simulink model "AMCLIB_CurrentLoop_BAM_FLT"  (Simulink 8.3)
settings: Solver=ode45  StartTime=0.0  StopTime=10.0  RelTol=1e-3
undefined symbols (not defined in the file): fltCC1scD, fltCC1scQ, fltCC2scD, fltCC2scQ
settings Model: Creator=B37097  LastModifiedBy=B37097
settings DataIOCC: SignalLoggingSaveFormat=Dataset
settings DebuggingCC: UnderspecifiedInitializationDetection=Simplified  StateNameClashWarn=none
settings GRTTargetCC: CombineOutputUpdateFcns=on  GRTInterface=off

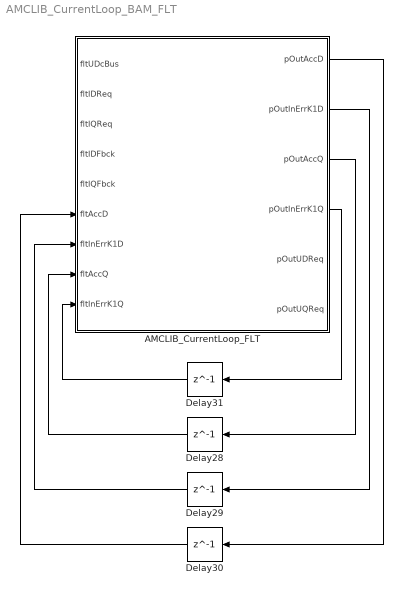
== system AMCLIB_CurrentLoop_BAM_FLT ==
  AMCLIB_CurrentLoop_FLT : Subsystem  mask(AMCLIB_CurrentLoop_FLT){fltCC1scD=fltCC1scD, fltCC2scD=fltCC2scD, fltCC1scQ=fltCC1scQ, fltCC2scQ=fltCC2scQ}
      mask help: Bit accurate model of the current loop algorithm for a PMSM. All parameters as well as input and output values are in single precision floating data format.
      mask init:
      | pos = get_param(gcb, 'Position');width = pos(3) - pos(1); height = pos(4) - pos(2);tX=width/2;tY=height*0.9;
      mask Display: color('black');port_label('input',1,'fltUDcBus');port_label('input',2,'fltIDReq');port_label('input',3,'fltIQReq');port_label('input',4,'fltIDFbck');port_label('input',5,'fltIQFbck');port_label('input',6,'fltAccD');port_label('input',7,'fltInErrK1D');port_label('input',8,'fltAccQ');port_label('input',9,'fltInErrK1Q');port_label('output',1,'pOutAccD');port_label('output',2,'pOutInErrK1D');port_label('output',3,'pOutAccQ');port_label('output',4,'pOutInErrK1Q');port_label('output',5,'pOutUDReq');port_label('output',6,'pOutUQReq');color('black');disp('AMCLIB_CurrentLoop_FLT');color('blue');text(tX,tY, 'BAM', 'horizontalAlignment', 'center');
  Delay{28..31} (4 alike) : Delay  DelayLength=1  InitialCondition=0
  wires:
  AMCLIB_CurrentLoop_FLT/4(pOutInErrK1Q) -> Delay31/1
  Delay31/1 -> AMCLIB_CurrentLoop_FLT/9(fltInErrK1Q)
  AMCLIB_CurrentLoop_FLT/3(pOutAccQ) -> Delay28/1
  Delay28/1 -> AMCLIB_CurrentLoop_FLT/8(fltAccQ)
  AMCLIB_CurrentLoop_FLT/2(pOutInErrK1D) -> Delay29/1
  Delay29/1 -> AMCLIB_CurrentLoop_FLT/7(fltInErrK1D)
  AMCLIB_CurrentLoop_FLT/1(pOutAccD) -> Delay30/1
  Delay30/1 -> AMCLIB_CurrentLoop_FLT/6(fltAccD)

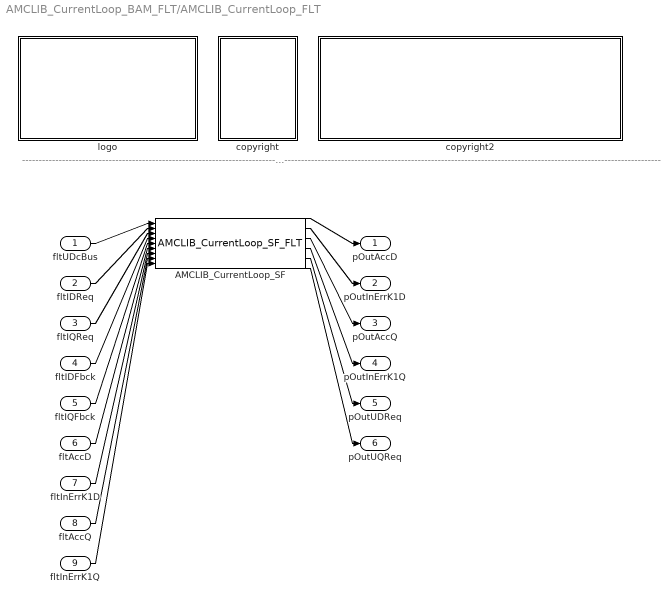
== system AMCLIB_CurrentLoop_BAM_FLT/AMCLIB_CurrentLoop_FLT ==
  note: ---------------------------------------------------------------------------------------------------------------------------------------------------------------------------------------------------
  fltUDcBus : Inport
  fltIDReq : Inport  Port=2
  fltIQReq : Inport  Port=3
  fltIDFbck : Inport  Port=4
  fltIQFbck : Inport  Port=5
  fltAccD : Inport  Port=6
  fltInErrK1D : Inport  Port=7
  fltAccQ : Inport  Port=8
  fltInErrK1Q : Inport  Port=9
  AMCLIB_CurrentLoop_SF : S-Function  FunctionName=AMCLIB_CurrentLoop_SF_FLT  Parameters=fltCC1scD,fltCC2scD,fltCC1scQ,fltCC2scQ  EnableBusSupport=off
  copyright : Subsystem
      mask Display: text(10,90,'FILE:');text(10,75,'DESRIPTION:');text(10,60,'COPYRIGHT:');text(10,45,'VERSION:');text(10,30,'DATE:')
  copyright2 : Subsystem
      mask Display: text(10,90,'AMCLIB_CurrentLoop_BAM_FLT.mdl');text(10,75,'PMSM Current Loop.');text(10,60,'NXP');text(10,45,'1.0');text(10,30,'25-Oct-2017');
  logo : Subsystem
      mask Display: image(imread('logo.jpg'))
  pOutAccD : Outport
  pOutInErrK1D : Outport  Port=2
  pOutAccQ : Outport  Port=3
  pOutInErrK1Q : Outport  Port=4
  pOutUDReq : Outport  Port=5
  pOutUQReq : Outport  Port=6
  wires:
  fltUDcBus/1 -> AMCLIB_CurrentLoop_SF/1
  fltIDReq/1 -> AMCLIB_CurrentLoop_SF/2
  fltIQReq/1 -> AMCLIB_CurrentLoop_SF/3
  fltIDFbck/1 -> AMCLIB_CurrentLoop_SF/4
  fltIQFbck/1 -> AMCLIB_CurrentLoop_SF/5
  fltAccD/1 -> AMCLIB_CurrentLoop_SF/6
  fltInErrK1D/1 -> AMCLIB_CurrentLoop_SF/7
  fltAccQ/1 -> AMCLIB_CurrentLoop_SF/8
  fltInErrK1Q/1 -> AMCLIB_CurrentLoop_SF/9
  AMCLIB_CurrentLoop_SF/1 -> pOutAccD/1
  AMCLIB_CurrentLoop_SF/2 -> pOutInErrK1D/1
  AMCLIB_CurrentLoop_SF/3 -> pOutAccQ/1
  AMCLIB_CurrentLoop_SF/4 -> pOutInErrK1Q/1
  AMCLIB_CurrentLoop_SF/5 -> pOutUDReq/1
  AMCLIB_CurrentLoop_SF/6 -> pOutUQReq/1

== system AMCLIB_CurrentLoop_BAM_FLT/AMCLIB_CurrentLoop_FLT/copyright ==

== system AMCLIB_CurrentLoop_BAM_FLT/AMCLIB_CurrentLoop_FLT/copyright2 ==

== system AMCLIB_CurrentLoop_BAM_FLT/AMCLIB_CurrentLoop_FLT/logo ==
